simulink model "TST_EGRVlv_DD"  (R2016b)
settings: Solver=FixedStepDiscrete  StartTime=0.0  StopTime=simTime  FixedStep=sampleTime  RelTol=1e-3
values from neighbouring files (symbols this model uses):
  testCase = 1    [initTST_EGRVlv_DD_001.m]
libraries: simulink x5, UnitTest_Lib x3
settings Model: Creator=zhulinfeng  LastModifiedBy=zhulinfeng
settings DebuggingCC: SignalRangeChecking=error

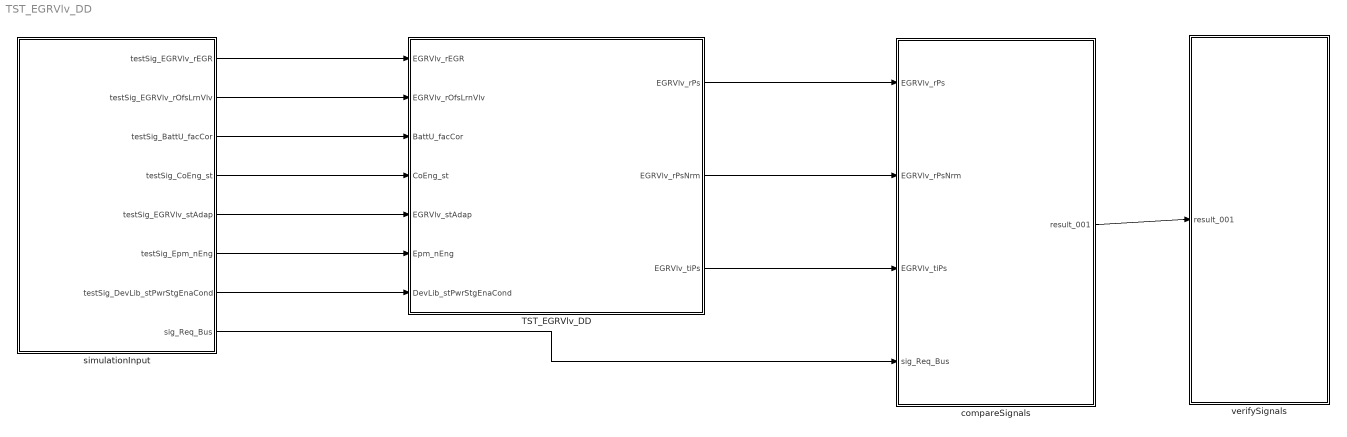
== system TST_EGRVlv_DD ==
  TST_EGRVlv_DD : Subsystem
  compareSignals : Subsystem
  simulationInput : Subsystem
  verifySignals : Subsystem
  wires:
  simulationInput/1(testSig_EGRVlv_rEGR) -> TST_EGRVlv_DD/1(EGRVlv_rEGR)
  simulationInput/2(testSig_EGRVlv_rOfsLrnVlv) -> TST_EGRVlv_DD/2(EGRVlv_rOfsLrnVlv)
  simulationInput/3(testSig_BattU_facCor) -> TST_EGRVlv_DD/3(BattU_facCor)
  simulationInput/4(testSig_CoEng_st) -> TST_EGRVlv_DD/4(CoEng_st)
  simulationInput/5(testSig_EGRVlv_stAdap) -> TST_EGRVlv_DD/5(EGRVlv_stAdap)
  simulationInput/6(testSig_Epm_nEng) -> TST_EGRVlv_DD/6(Epm_nEng)
  simulationInput/7(testSig_DevLib_stPwrStgEnaCond) -> TST_EGRVlv_DD/7(DevLib_stPwrStgEnaCond)
  TST_EGRVlv_DD/1(EGRVlv_rPs) -> compareSignals/1(EGRVlv_rPs)
  TST_EGRVlv_DD/2(EGRVlv_rPsNrm) -> compareSignals/2(EGRVlv_rPsNrm)
  TST_EGRVlv_DD/3(EGRVlv_tiPs) -> compareSignals/3(EGRVlv_tiPs)
  simulationInput/8(sig_Req_Bus) -> compareSignals/4(sig_Req_Bus)
  compareSignals/1(result_001) -> verifySignals/1(result_001)

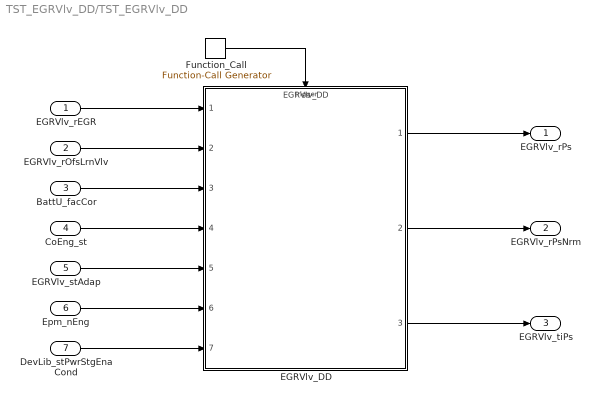
== system TST_EGRVlv_DD/TST_EGRVlv_DD ==
  EGRVlv_rEGR : Inport
  EGRVlv_rOfsLrnVlv : Inport  Port=2
  BattU_facCor : Inport  Port=3
  CoEng_st : Inport  Port=4
  EGRVlv_stAdap : Inport  Port=5
  Epm_nEng : Inport  Port=6
  DevLib_stPwrStgEnaCond : Inport  Port=7
  EGRVlv_DD : ModelReference  ModelNameDialog=EGRVlv_DD  SimulationMode=Normal  ModelReferenceVersion=1.20  TriggerPortName=function  TriggerPortTriggerType=function-call  TriggerPortStatesWhenEnabling=held
  Function_Call : simulink/Ports & Subsystems/Function-Call Generator  sample_time=sampleTime  numberOfIterations=1
  EGRVlv_rPs : Outport
  EGRVlv_rPsNrm : Outport  Port=2
  EGRVlv_tiPs : Outport  Port=3
  wires:
  Function_Call/1 -> EGRVlv_DD/Trigger
  EGRVlv_rEGR/1 -> EGRVlv_DD/1
  EGRVlv_rOfsLrnVlv/1 -> EGRVlv_DD/2
  BattU_facCor/1 -> EGRVlv_DD/3
  CoEng_st/1 -> EGRVlv_DD/4
  EGRVlv_stAdap/1 -> EGRVlv_DD/5
  Epm_nEng/1 -> EGRVlv_DD/6
  DevLib_stPwrStgEnaCond/1 -> EGRVlv_DD/7
  EGRVlv_DD/1 -> EGRVlv_rPs/1
  EGRVlv_DD/2 -> EGRVlv_rPsNrm/1
  EGRVlv_DD/3 -> EGRVlv_tiPs/1

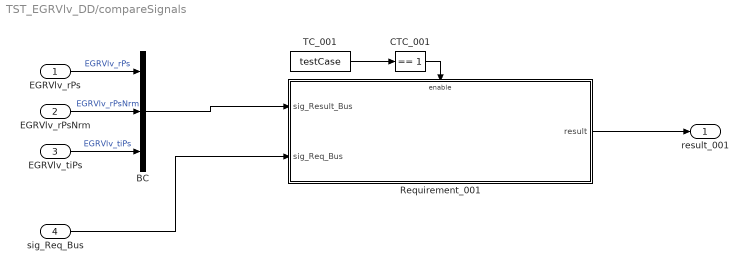
== system TST_EGRVlv_DD/compareSignals ==
  EGRVlv_rPs : Inport
  EGRVlv_rPsNrm : Inport  Port=2
  EGRVlv_tiPs : Inport  Port=3
  sig_Req_Bus : Inport  Port=4
  BC : BusCreator  Inputs=3
  CTC_001 : simulink/Logic and Bit Operations/Compare To Constant  relop===  const=1  OutDataTypeStr=boolean
  Requirement_001 : Subsystem
  TC_001 : Constant  Value=testCase
  result_001 : Outport
  wires:
  EGRVlv_rPs/1 -> BC/1  "EGRVlv_rPs"
  EGRVlv_rPsNrm/1 -> BC/2  "EGRVlv_rPsNrm"
  EGRVlv_tiPs/1 -> BC/3  "EGRVlv_tiPs"
  TC_001/1 -> CTC_001/1
  CTC_001/1 -> Requirement_001/Enable
  sig_Req_Bus/1 -> Requirement_001/2(sig_Req_Bus)
  BC/1 -> Requirement_001/1(sig_Result_Bus)
  Requirement_001/1(result) -> result_001/1

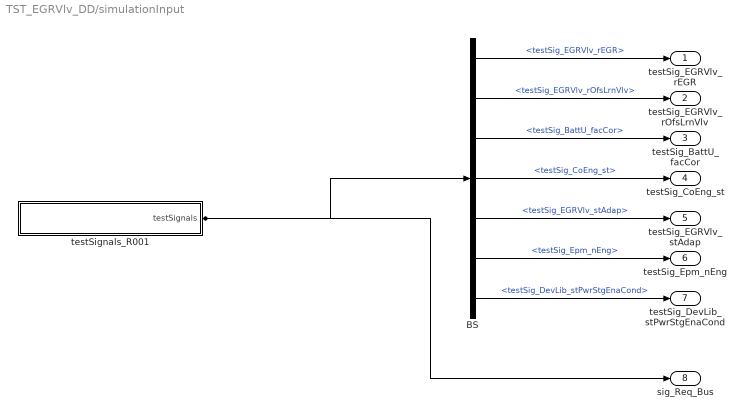
== system TST_EGRVlv_DD/simulationInput ==
  BS : BusSelector  OutputSignals=testSig_EGRVlv_rEGR,testSig_EGRVlv_rOfsLrnVlv,testSig_BattU_facCor,testSig_CoEng_st,testSig_EGRVlv_stAdap,testSig_Epm_nEng,testSig_DevLib_stPwrStgEnaCond
  testSignals_R001 : Subsystem
  testSig_EGRVlv_rEGR : Outport
  testSig_EGRVlv_rOfsLrnVlv : Outport  Port=2
  testSig_BattU_facCor : Outport  Port=3
  testSig_CoEng_st : Outport  Port=4
  testSig_EGRVlv_stAdap : Outport  Port=5
  testSig_Epm_nEng : Outport  Port=6
  testSig_DevLib_stPwrStgEnaCond : Outport  Port=7
  sig_Req_Bus : Outport  Port=8
  wires:
  BS/1 -> testSig_EGRVlv_rEGR/1  "<testSig_EGRVlv_rEGR>"
  BS/2 -> testSig_EGRVlv_rOfsLrnVlv/1  "<testSig_EGRVlv_rOfsLrnVlv>"
  BS/3 -> testSig_BattU_facCor/1  "<testSig_BattU_facCor>"
  BS/4 -> testSig_CoEng_st/1  "<testSig_CoEng_st>"
  BS/5 -> testSig_EGRVlv_stAdap/1  "<testSig_EGRVlv_stAdap>"
  BS/6 -> testSig_Epm_nEng/1  "<testSig_Epm_nEng>"
  BS/7 -> testSig_DevLib_stPwrStgEnaCond/1  "<testSig_DevLib_stPwrStgEnaCond>"
  testSignals_R001/1(testSignals) -> BS/1, sig_Req_Bus/1

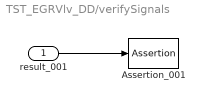
== system TST_EGRVlv_DD/verifySignals ==
  result_001 : Inport
  Assertion_001 : Assertion  Enabled=off
  wires:
  result_001/1 -> Assertion_001/1

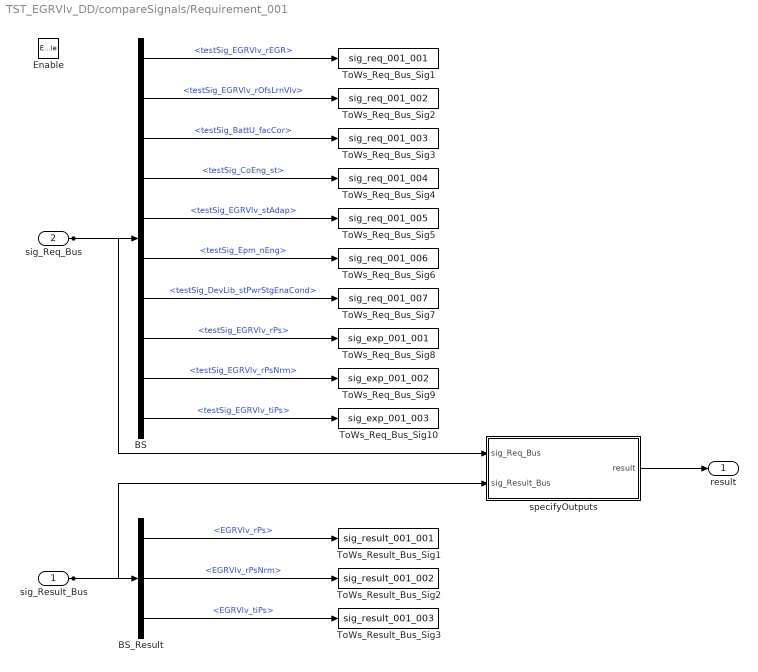
== system TST_EGRVlv_DD/compareSignals/Requirement_001 ==
  sig_Result_Bus : Inport
  sig_Req_Bus : Inport  Port=2
  Enable : EnablePort
  BS : BusSelector  OutputSignals=testSig_EGRVlv_rEGR,testSig_EGRVlv_rOfsLrnVlv,testSig_BattU_facCor,testSig_CoEng_st,testSig_EGRVlv_stAdap,testSig_Epm_nEng,testSig_DevLib_stPwrStgEnaCond,testSig_EGRVlv_rPs,testSig_EGRVlv_rPsNrm,testSig_EGRVlv_tiPs
  BS_Result : BusSelector  OutputSignals=EGRVlv_rPs,EGRVlv_rPsNrm,EGRVlv_tiPs
  ToWs_Req_Bus_Sig1 : ToWorkspace  VariableName=sig_req_001_001  SaveFormat=Structure With Time
  ToWs_Req_Bus_Sig10 : ToWorkspace  VariableName=sig_exp_001_003  SaveFormat=Structure With Time
  ToWs_Req_Bus_Sig2 : ToWorkspace  VariableName=sig_req_001_002  SaveFormat=Structure With Time
  ToWs_Req_Bus_Sig3 : ToWorkspace  VariableName=sig_req_001_003  SaveFormat=Structure With Time
  ToWs_Req_Bus_Sig4 : ToWorkspace  VariableName=sig_req_001_004  SaveFormat=Structure With Time
  ToWs_Req_Bus_Sig5 : ToWorkspace  VariableName=sig_req_001_005  SaveFormat=Structure With Time
  ToWs_Req_Bus_Sig6 : ToWorkspace  VariableName=sig_req_001_006  SaveFormat=Structure With Time
  ToWs_Req_Bus_Sig7 : ToWorkspace  VariableName=sig_req_001_007  SaveFormat=Structure With Time
  ToWs_Req_Bus_Sig8 : ToWorkspace  VariableName=sig_exp_001_001  SaveFormat=Structure With Time
  ToWs_Req_Bus_Sig9 : ToWorkspace  VariableName=sig_exp_001_002  SaveFormat=Structure With Time
  ToWs_Result_Bus_Sig1 : ToWorkspace  VariableName=sig_result_001_001  SaveFormat=Structure With Time
  ToWs_Result_Bus_Sig2 : ToWorkspace  VariableName=sig_result_001_002  SaveFormat=Structure With Time
  ToWs_Result_Bus_Sig3 : ToWorkspace  VariableName=sig_result_001_003  SaveFormat=Structure With Time
  specifyOutputs : Subsystem
  result : Outport
  wires:
  sig_Req_Bus/1 -> BS/1, specifyOutputs/1(sig_Req_Bus)
  BS/1 -> ToWs_Req_Bus_Sig1/1  "<testSig_EGRVlv_rEGR>"
  BS/2 -> ToWs_Req_Bus_Sig2/1  "<testSig_EGRVlv_rOfsLrnVlv>"
  BS/3 -> ToWs_Req_Bus_Sig3/1  "<testSig_BattU_facCor>"
  BS/4 -> ToWs_Req_Bus_Sig4/1  "<testSig_CoEng_st>"
  BS/5 -> ToWs_Req_Bus_Sig5/1  "<testSig_EGRVlv_stAdap>"
  BS/6 -> ToWs_Req_Bus_Sig6/1  "<testSig_Epm_nEng>"
  BS/7 -> ToWs_Req_Bus_Sig7/1  "<testSig_DevLib_stPwrStgEnaCond>"
  BS/8 -> ToWs_Req_Bus_Sig8/1  "<testSig_EGRVlv_rPs>"
  BS/9 -> ToWs_Req_Bus_Sig9/1  "<testSig_EGRVlv_rPsNrm>"
  BS/10 -> ToWs_Req_Bus_Sig10/1  "<testSig_EGRVlv_tiPs>"
  sig_Result_Bus/1 -> BS_Result/1, specifyOutputs/2(sig_Result_Bus)
  BS_Result/1 -> ToWs_Result_Bus_Sig1/1  "<EGRVlv_rPs>"
  BS_Result/2 -> ToWs_Result_Bus_Sig2/1  "<EGRVlv_rPsNrm>"
  BS_Result/3 -> ToWs_Result_Bus_Sig3/1  "<EGRVlv_tiPs>"
  specifyOutputs/1(result) -> result/1

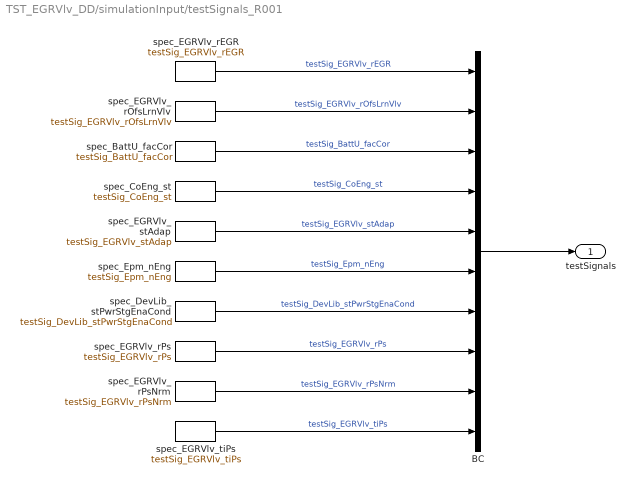
== system TST_EGRVlv_DD/simulationInput/testSignals_R001 ==
  BC : BusCreator  Inputs=10
  spec_BattU_facCor : FromWorkspace  VariableName=testSig_BattU_facCor  Interpolate=off  OutputAfterFinalValue=Holding final value
  spec_CoEng_st : FromWorkspace  VariableName=testSig_CoEng_st  Interpolate=off  OutputAfterFinalValue=Holding final value
  spec_DevLib_stPwrStgEnaCond : FromWorkspace  VariableName=testSig_DevLib_stPwrStgEnaCond  Interpolate=off  OutputAfterFinalValue=Holding final value
  spec_EGRVlv_rEGR : FromWorkspace  VariableName=testSig_EGRVlv_rEGR  Interpolate=off  OutputAfterFinalValue=Holding final value
  spec_EGRVlv_rOfsLrnVlv : FromWorkspace  VariableName=testSig_EGRVlv_rOfsLrnVlv  Interpolate=off  OutputAfterFinalValue=Holding final value
  spec_EGRVlv_rPs : FromWorkspace  VariableName=testSig_EGRVlv_rPs  Interpolate=off  OutputAfterFinalValue=Holding final value
  spec_EGRVlv_rPsNrm : FromWorkspace  VariableName=testSig_EGRVlv_rPsNrm  Interpolate=off  OutputAfterFinalValue=Holding final value
  spec_EGRVlv_stAdap : FromWorkspace  VariableName=testSig_EGRVlv_stAdap  Interpolate=off  OutputAfterFinalValue=Holding final value
  spec_EGRVlv_tiPs : FromWorkspace  VariableName=testSig_EGRVlv_tiPs  Interpolate=off  OutputAfterFinalValue=Holding final value
  spec_Epm_nEng : FromWorkspace  VariableName=testSig_Epm_nEng  Interpolate=off  OutputAfterFinalValue=Holding final value
  testSignals : Outport
  wires:
  BC/1 -> testSignals/1
  spec_EGRVlv_rEGR/1 -> BC/1  "testSig_EGRVlv_rEGR"
  spec_EGRVlv_rOfsLrnVlv/1 -> BC/2  "testSig_EGRVlv_rOfsLrnVlv"
  spec_BattU_facCor/1 -> BC/3  "testSig_BattU_facCor"
  spec_CoEng_st/1 -> BC/4  "testSig_CoEng_st"
  spec_EGRVlv_stAdap/1 -> BC/5  "testSig_EGRVlv_stAdap"
  spec_Epm_nEng/1 -> BC/6  "testSig_Epm_nEng"
  spec_DevLib_stPwrStgEnaCond/1 -> BC/7  "testSig_DevLib_stPwrStgEnaCond"
  spec_EGRVlv_rPs/1 -> BC/8  "testSig_EGRVlv_rPs"
  spec_EGRVlv_rPsNrm/1 -> BC/9  "testSig_EGRVlv_rPsNrm"
  spec_EGRVlv_tiPs/1 -> BC/10  "testSig_EGRVlv_tiPs"

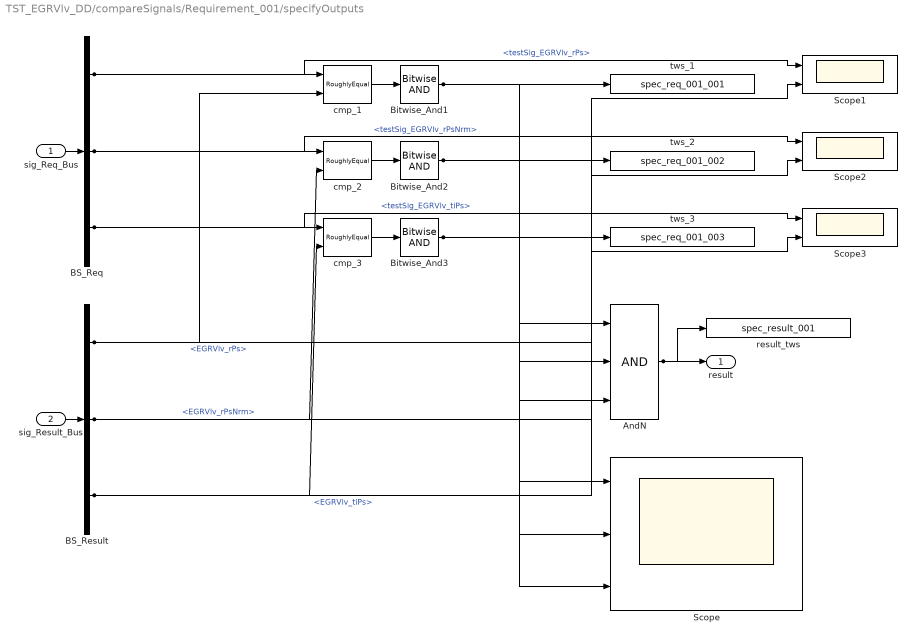
== system TST_EGRVlv_DD/compareSignals/Requirement_001/specifyOutputs ==
  sig_Req_Bus : Inport
  sig_Result_Bus : Inport  Port=2
  AndN : Logic  Inputs=3
  BS_Req : BusSelector  OutputSignals=testSig_EGRVlv_rPs,testSig_EGRVlv_rPsNrm,testSig_EGRVlv_tiPs
  BS_Result : BusSelector  OutputSignals=EGRVlv_rPs,EGRVlv_rPsNrm,EGRVlv_tiPs
  Bitwise_And1 : simulink/Logic and Bit Operations/Bitwise Operator  logicop=AND  UseBitMask=off  BitMask=bin2dec('11011001')  BitMaskRealWorld=Stored Integer
  Bitwise_And2 : simulink/Logic and Bit Operations/Bitwise Operator  logicop=AND  UseBitMask=off  BitMask=bin2dec('11011001')  BitMaskRealWorld=Stored Integer
  Bitwise_And3 : simulink/Logic and Bit Operations/Bitwise Operator  logicop=AND  UseBitMask=off  BitMask=bin2dec('11011001')  BitMaskRealWorld=Stored Integer
  Scope : Scope  NumInputPorts=3
  Scope1 : Scope  NumInputPorts=2
  Scope2 : Scope  NumInputPorts=2
  Scope3 : Scope  NumInputPorts=2
  cmp_1 : UnitTest_Lib/RoughlyEqual  slope=0.1
  cmp_2 : UnitTest_Lib/RoughlyEqual  slope=0.1
  cmp_3 : UnitTest_Lib/RoughlyEqual  slope=0.1
  result_tws : ToWorkspace  VariableName=spec_result_001
  tws_1 : ToWorkspace  VariableName=spec_req_001_001
  tws_2 : ToWorkspace  VariableName=spec_req_001_002
  tws_3 : ToWorkspace  VariableName=spec_req_001_003
  result : Outport
  wires:
  sig_Req_Bus/1 -> BS_Req/1
  sig_Result_Bus/1 -> BS_Result/1
  AndN/1 -> result/1, result_tws/1
  BS_Req/1 -> cmp_1/1, Scope1/1  "<testSig_EGRVlv_rPs>"
  BS_Result/1 -> cmp_1/2, Scope1/2  "<EGRVlv_rPs>"
  cmp_1/1 -> Bitwise_And1/1
  Bitwise_And1/1 -> tws_1/1, AndN/1, Scope/1
  BS_Req/2 -> cmp_2/1, Scope2/1  "<testSig_EGRVlv_rPsNrm>"
  BS_Result/2 -> cmp_2/2, Scope2/2  "<EGRVlv_rPsNrm>"
  cmp_2/1 -> Bitwise_And2/1
  Bitwise_And2/1 -> tws_2/1, AndN/2, Scope/2
  BS_Req/3 -> cmp_3/1, Scope3/1  "<testSig_EGRVlv_tiPs>"
  BS_Result/3 -> cmp_3/2, Scope3/2  "<EGRVlv_tiPs>"
  cmp_3/1 -> Bitwise_And3/1
  Bitwise_And3/1 -> tws_3/1, AndN/3, Scope/3
